simulink model "Question_1"  (R2024b)
settings: Solver=VariableStepAuto  StartTime=0.0  StopTime=10.0  RelTol=1e-3
model workspace (MAT data in the model file):
  a = 16
  b = 6
  choice = 2
settings Model: Creator=Sagar  LastModifiedBy=Sagar

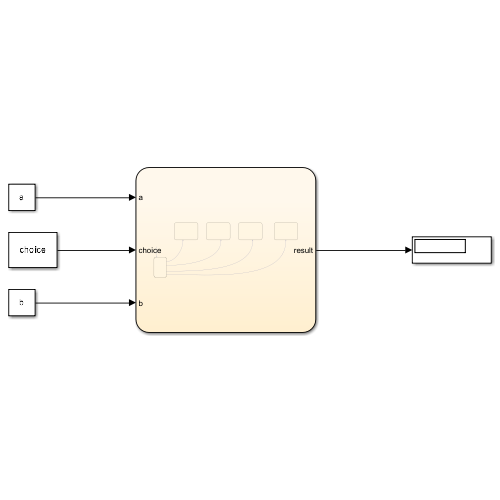
[thumbnail: Simulink's stored preview of the top-level diagram]
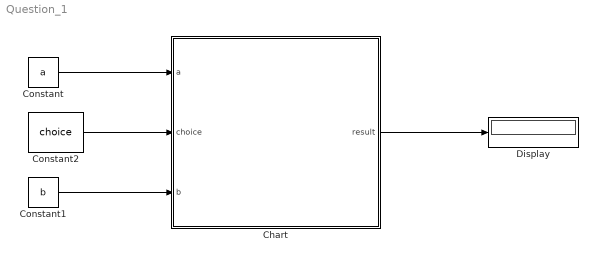
== system Question_1 ==
  Chart : Stateflow chart  TreatAsAtomicUnit=on
  Constant : Constant  Value=a
  Constant1 : Constant  Value=b
  Constant2 : Constant  Value=choice
  Display : Display
  wires:
  Constant/1 -> Chart/1(a)
  Constant1/1 -> Chart/3(b)
  Constant2/1 -> Chart/2(choice)
  Chart/1(result) -> Display/1

== stateflow chart Question_1/Chart ==
  state Addition
    entry:
    result=a+b
  state Subtraction
    entry:
    result=a-b
  state Multiplication
    entry:
    result=a*b
  state Division
    entry:
    result=a/b;
  state Choice
  Choice -> Multiplication [order 4] : [choice == 3]
  Choice -> Subtraction [order 3] : [choice == 2]
  Choice -> Addition [order 2] : [choice == 1]
  Choice -> Division [order 1] : [choice ==4 ]
  (default) -> Choice
  data: a input; choice input; b input; result output
